simulink model "Vaxelriktare_Transducers"  (R2020b)
settings: Solver=VariableStepAuto  StartTime=0.0  StopTime=0.01  RelTol=1e-3
libraries: fl_lib x80, nesl_utility x32, ee_lib x3, SignalEditorBlockLib x1
(part 2 of 2)

== system Vaxelriktare_Transducers/Temperature transducer/0.76 V from voltage divider ==
  Constant : Constant  Value=0.76
  Controlled Voltage Source1 : fl_lib/Electrical/Electrical Sources/Controlled Voltage Source
  Electrical Reference3 : fl_lib/Electrical/Electrical Elements/Electrical Reference
  Simulink-PS Converter1 : nesl_utility/Simulink-PS Converter  PhysicalDomain=network_engine_domain  SubClassName=ps_input  LeftPortType=input  RightPortType=output  PseudoPeriodic=off  Frequencies=[]  NoiseDistribution=none  NoiseParameters=[]  Unit=1  AffineConversion=off  FilteringAndDerivatives=provide  SimscapeFilterOrder=1  InputFilterTimeConstant=0.001  UdotUserProvided=0
  Controlled Voltage Source2 : PMIOPort  Side=Right
  wires:
  Constant/1 -> Simulink-PS Converter1/1
  connections:
  Simulink-PS Converter1/RConn1 -- Controlled Voltage Source1/RConn1
  Electrical Reference3/LConn1 -- Controlled Voltage Source1/RConn2
  Controlled Voltage Source2/RConn1 -- Controlled Voltage Source1/LConn1

== system Vaxelriktare_Transducers/Temperature transducer/LM35 ==
  Temperature : Inport
  Electrical Reference1 : fl_lib/Electrical/Electrical Elements/Electrical Reference
  Gain : Gain  Gain=1/100
  LM35 : fl_lib/Electrical/Electrical Sources/Controlled Voltage Source
  Simulink-PS Converter3 : nesl_utility/Simulink-PS Converter  PhysicalDomain=network_engine_domain  SubClassName=ps_input  LeftPortType=input  RightPortType=output  PseudoPeriodic=off  Frequencies=[]  NoiseDistribution=none  NoiseParameters=[]  Unit=1  AffineConversion=off  FilteringAndDerivatives=provide  SimscapeFilterOrder=1  InputFilterTimeConstant=0.001  UdotUserProvided=0
  Controlled Voltage Source1 : PMIOPort  Side=Right
  wires:
  Gain/1 -> Simulink-PS Converter3/1
  Temperature/1 -> Gain/1
  connections:
  LM35/LConn1 -- Controlled Voltage Source1/RConn1
  Simulink-PS Converter3/RConn1 -- LM35/RConn1
  Electrical Reference1/LConn1 -- LM35/RConn2
